simulink model "sampleModel184"  (R2021b)
settings: Solver=VariableStepAuto  StartTime=0.0  StopTime=10.0  RelTol=1e-3
libraries: simulink x11
settings Model: Creator=user  LastModifiedBy=user

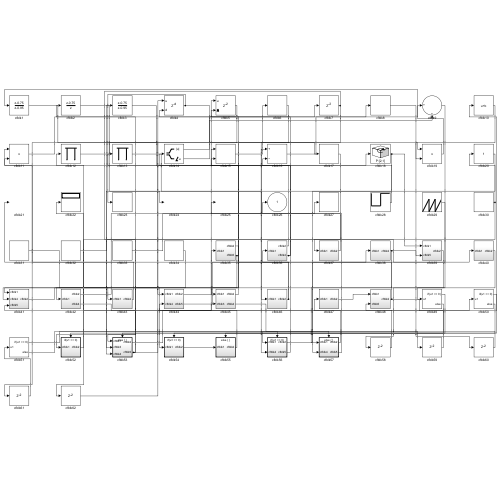
[thumbnail: Simulink's stored preview of the top-level diagram]
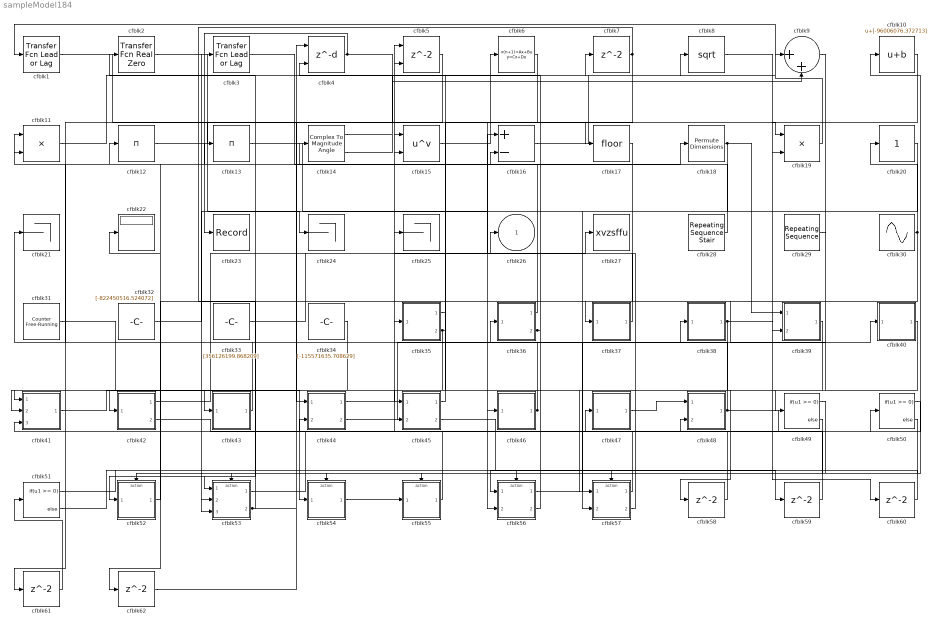
== system sampleModel184 ==
  cfblk1 : simulink/Discrete/Transfer Fcn Lead or Lag  PoleZ=0.95  ZeroZ=0.75  ICPrevOutput=0.0  ICPrevInput=0.0  DoSatur=off
      settings: SourceProductBaseCode=SL
  cfblk10 : Bias  Bias=[-96006076.372713]
  cfblk11 : Product  Inputs=**
  cfblk12 : Product  Inputs=*
  cfblk13 : Product  Inputs=*
  cfblk14 : ComplexToMagnitudeAngle
  cfblk15 : Math  Operator=pow  SaturateOnIntegerOverflow=on
  cfblk16 : Sum  Inputs=+-
  cfblk17 : Rounding
  cfblk18 : PermuteDimensions
  cfblk19 : Product
  cfblk2 : simulink/Discrete/Transfer Fcn Real Zero  ZeroZ=0.75  ICPrevInput=0.0  DoSatur=off
      settings: SourceProductBaseCode=SL
  cfblk20 : simulink/Math Operations/Slider Gain  gain=1  low=0  high=2
  cfblk21 : Terminator
  cfblk22 : Display
  cfblk23 : Record  FileSettingsInternal="{\"entries\":[{\"content\":{\"excelSettings\":{\"content\":{},\"type\":\"Streamout.ExcelSettings\"}},\"type\":\"Streamout.FileSettingStorage\",\"uuid\":\"3bb29845-961e-4fee-bd6d-4ce92e24b57c\"}],\"packageUris\":[\"http://schema.mathworks.com/mf0/streamout_blocks/R2020a\"],\"version\":\"1.0\"}"  SignalsInternal="{\"entries\":[{\"content\":{\"signals\":[{\"content\":{\"blockPath\":[\"sampleModel184/cfblk23\"],\"channel\":[],\"dimensions\":[1],\"domain\":\"sampleModel184/cfblk23\",\"lineColor\":\"#4dbeee\",\"plots\":[1],\"port\":1,\"sid\":[\"\"],\"signalID\":6859,\"signalName\":\"cfblk4\"},\"type\":\"RecordBlkView.Signal\",\"uuid\":\"63a490c9-4ba1-4137-91fe-6ad1500206e2\"}]},\"type\":\"RecordBlkView.InputSignals\",\"uuid\":\"3eea0c6d-d5bb-49b1-9db6-edc089c19657\"}],\"packageUris\":[\"http://schema.mathworks.com/mf0/streamout_blocks/R2020a\"],\"version\":\"1.0\"}"  VisualizationBindings="{\"sparklinesplugin\":{\"info\":[{\"bindingParametersList\":[],\"subplotID\":1}]}}"
  cfblk24 : Terminator
  cfblk25 : Terminator
  cfblk27 : ToWorkspace  VariableName=xvzsffu  SaveFormat=Timeseries  SampleTime=-1
  cfblk28 : simulink/Sources/Repeating Sequence Stair  OutValues=[100473429.883749, 716274051.172989]  tsamp=-1  OutMin=[]  OutMax=[]  OutDataTypeStr=double  OutputDataTypeScalingMode=double  OutDataType=fixdt(0,8)  ConRadixGroup=Best Precision: Vector-wise  OutScaling=2^-12
  cfblk29 : simulink/Sources/Repeating Sequence  rep_seq_t=[0 2]  rep_seq_y=[-291271804.102666, -101111727.446018]
  cfblk3 : simulink/Discrete/Transfer Fcn Lead or Lag  PoleZ=0.95  ZeroZ=0.75  ICPrevOutput=0.0  ICPrevInput=0.0  DoSatur=off
      settings: SourceProductBaseCode=SL
  cfblk30 : Sin  Amplitude=[486537178.471700]  Bias=[-87359593.712021]  SampleTime=0
  cfblk31 : simulink/Sources/Counter Free-Running  NumBits=[28.000000]  tsamp=-1
  cfblk32 : Constant  Value=[-822450516.524072]  SampleTime=1
  cfblk33 : Constant  Value=[356126199.868209]  SampleTime=1
  cfblk34 : Constant  Value=[-115571635.708629]  SampleTime=1
  cfblk35 : Subsystem
  cfblk36 : Subsystem
  cfblk37 : Subsystem
  cfblk38 : Subsystem
  cfblk39 : Subsystem
  cfblk4 : Delay  DelayLengthSource=Input port  SampleTime=1
      settings: InputPortMap=u0,p1
  cfblk40 : Subsystem
  cfblk41 : Subsystem
  cfblk42 : Subsystem
  cfblk43 : Subsystem
  cfblk44 : Subsystem
  cfblk45 : Subsystem
  cfblk46 : Subsystem
  cfblk47 : Subsystem
  cfblk48 : Subsystem
  cfblk49 : If  IfExpression=u1 >= 0  SampleTime=1
  cfblk5 : Delay  ShowEnablePort=on  SampleTime=1
      settings: InputPortMap=u0,e6
  cfblk50 : If  IfExpression=u1 >= 0  SampleTime=1
  cfblk51 : If  IfExpression=u1 >= 0  SampleTime=1
  cfblk52 : Subsystem  TreatAsAtomicUnit=on
  cfblk53 : Subsystem  TreatAsAtomicUnit=on
  cfblk54 : Subsystem  TreatAsAtomicUnit=on
  cfblk55 : Subsystem  TreatAsAtomicUnit=on
  cfblk56 : Subsystem  TreatAsAtomicUnit=on
  cfblk57 : Subsystem  TreatAsAtomicUnit=on
  cfblk{7,58..62} (6 alike) : Delay  SampleTime=1
  cfblk6 : DiscreteStateSpace
  cfblk8 : Sqrt  SaturateOnIntegerOverflow=on
  cfblk9 : Sum  Inputs=|++
  cfblk26 : Outport
  wires:
  cfblk43/1(cfblk2) -> cfblk21/1
  cfblk54/1(cfblk2) -> cfblk55/1(cfblk1)
  cfblk4/1 -> cfblk23/1, cfblk17/1
  cfblk3/1 -> cfblk18/1
  cfblk30/1 -> cfblk20/1, cfblk53/3(cfblk4)
  cfblk18/1 -> cfblk39/1(cfblk1), cfblk53/2(cfblk3)
  cfblk57/1(cfblk2) -> cfblk47/1(cfblk1)
  cfblk7/1 -> cfblk52/1(cfblk1), cfblk45/1(cfblk1)
  cfblk2/1 -> cfblk24/1
  cfblk40/1(cfblk2) -> cfblk57/1(cfblk1)
  cfblk15/1 -> cfblk6/1
  cfblk38/1(cfblk2) -> cfblk60/1, cfblk61/1
  cfblk9/1 -> cfblk37/1(cfblk1)
  cfblk35/1(cfblk2) -> cfblk42/1(cfblk1)
  cfblk42/1(cfblk2) -> cfblk27/1
  cfblk48/1(cfblk2) -> cfblk10/1, cfblk11/2
  cfblk37/1(cfblk2) -> cfblk26/1
  cfblk56/1(cfblk2) -> cfblk38/1(cfblk1)
  cfblk44/1(cfblk2) -> cfblk5/1
  cfblk31/1 -> cfblk54/1(cfblk1)
  cfblk13/1 -> cfblk46/1(cfblk1)
  cfblk55/1(cfblk2) -> cfblk12/1
  cfblk12/1 -> cfblk19/1
  cfblk32/1 -> cfblk3/1
  cfblk52/1(cfblk2) -> cfblk22/1
  cfblk20/1 -> cfblk57/2(cfblk4)
  cfblk6/1 -> cfblk56/2(cfblk4)
  cfblk56/2(cfblk5) -> cfblk4/2
  cfblk41/1(cfblk2) -> cfblk43/1(cfblk1)
  cfblk8/1 -> cfblk19/2
  cfblk1/1 -> cfblk44/1(cfblk1)
  cfblk47/1(cfblk2) -> cfblk48/1(cfblk1)
  cfblk11/1 -> cfblk7/1
  cfblk19/1 -> cfblk1/1
  cfblk29/1 -> cfblk49/1
  cfblk42/2(cfblk4) -> cfblk50/1
  cfblk53/1(cfblk2) -> cfblk35/1(cfblk1)
  cfblk57/2(cfblk5) -> cfblk25/1
  cfblk33/1 -> cfblk16/1
  cfblk45/1(cfblk2) -> cfblk5/2
  cfblk16/1 -> cfblk8/1
  cfblk28/1 -> cfblk13/1
  cfblk35/2(cfblk5) -> cfblk15/1, cfblk41/2(cfblk4)
  cfblk34/1 -> cfblk53/1(cfblk1)
  cfblk53/2(cfblk5) -> cfblk2/1, cfblk41/3(cfblk5), cfblk45/2(cfblk3)
  cfblk10/1 -> cfblk39/2(cfblk5)
  cfblk46/1(cfblk2) -> cfblk36/1(cfblk1), cfblk15/2
  cfblk36/1(cfblk2) -> cfblk14/1
  cfblk44/2(cfblk5) -> cfblk40/1(cfblk1)
  cfblk36/2(cfblk4) -> cfblk16/2, cfblk11/1
  cfblk14/1 -> cfblk9/1
  cfblk5/1 -> cfblk41/1(cfblk1)
  cfblk14/2 -> cfblk9/2
  cfblk49/1 -> cfblk52/Action
  cfblk49/2 -> cfblk53/Action
  cfblk50/1 -> cfblk54/Action
  cfblk50/2 -> cfblk55/Action
  cfblk51/1 -> cfblk56/Action
  cfblk51/2 -> cfblk57/Action
  cfblk39/1(cfblk2) -> cfblk58/1
  cfblk58/1 -> cfblk48/2(cfblk5)
  cfblk45/2(cfblk4) -> cfblk59/1
  cfblk59/1 -> cfblk44/2(cfblk4)
  cfblk60/1 -> cfblk56/1(cfblk1)
  cfblk61/1 -> cfblk51/1
  cfblk17/1 -> cfblk62/1
  cfblk62/1 -> cfblk4/1

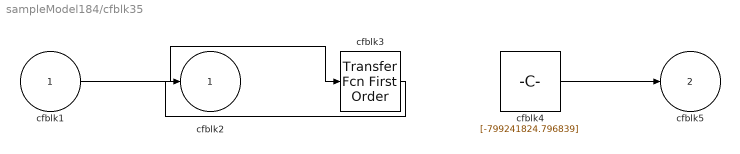
== system sampleModel184/cfblk35 ==
  cfblk1 : Inport
  cfblk3 : simulink/Discrete/Transfer Fcn First Order  PoleZ=0.95  ICPrevOutput=0.0  DoSatur=off
  cfblk4 : Constant  Value=[-799241824.796839]  SampleTime=1
  cfblk2 : Outport
  cfblk5 : Outport  Port=2
  wires:
  cfblk1/1 -> cfblk3/1
  cfblk4/1 -> cfblk5/1
  cfblk3/1 -> cfblk2/1

== system sampleModel184/cfblk36 ==
  cfblk1 : Inport
  cfblk3 : Assignment  DiagnosticForDimensions=Warning  IndexOptions=Index vector (dialog)  Indices=1  OutputSizes=1
  cfblk2 : Outport
  cfblk4 : Outport  Port=2
  wires:
  cfblk1/1 -> cfblk2/1, cfblk3/1, cfblk3/2
  cfblk3/1 -> cfblk4/1

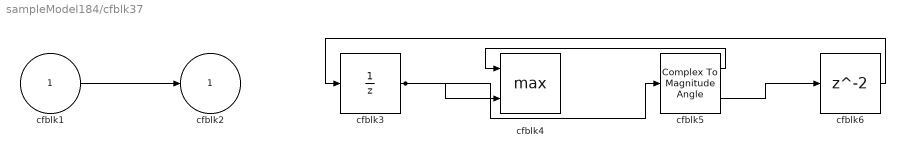
== system sampleModel184/cfblk37 ==
  cfblk1 : Inport
  cfblk3 : UnitDelay  HasFrameUpgradeWarning=on
  cfblk4 : MinMax  Function=max  Inputs=2
  cfblk5 : ComplexToMagnitudeAngle
  cfblk6 : Delay  SampleTime=1
  cfblk2 : Outport
  wires:
  cfblk1/1 -> cfblk2/1
  cfblk5/1 -> cfblk4/1
  cfblk3/1 -> cfblk5/1, cfblk4/2
  cfblk5/2 -> cfblk6/1
  cfblk6/1 -> cfblk3/1

== system sampleModel184/cfblk38 ==
  cfblk1 : Inport
  cfblk3 : ComplexToMagnitudeAngle
  cfblk4 : Bias  Bias=[821146582.759653]
  cfblk2 : Outport
  wires:
  cfblk3/1 -> cfblk2/1
  cfblk1/1 -> cfblk4/1
  cfblk4/1 -> cfblk3/1

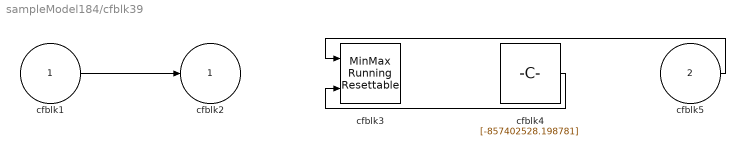
== system sampleModel184/cfblk39 ==
  cfblk1 : Inport
  cfblk5 : Inport  Port=2
  cfblk3 : simulink/Math Operations/MinMax Running Resettable  Function=min  vinit=0.0
  cfblk4 : Constant  Value=[-857402528.198781]  SampleTime=1
  cfblk2 : Outport
  wires:
  cfblk1/1 -> cfblk2/1
  cfblk5/1 -> cfblk3/1
  cfblk4/1 -> cfblk3/2

== system sampleModel184/cfblk40 ==
  cfblk1 : Inport
  cfblk3 : Constant  Value=[639037280.351687]  SampleTime=1
  cfblk2 : Outport
  wires:
  cfblk1/1 -> cfblk2/1

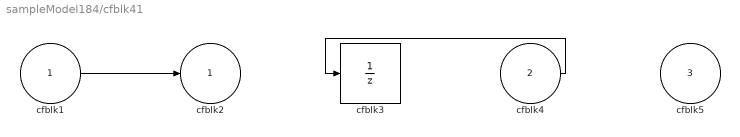
== system sampleModel184/cfblk41 ==
  cfblk1 : Inport
  cfblk4 : Inport  Port=2
  cfblk5 : Inport  Port=3
  cfblk3 : UnitDelay  HasFrameUpgradeWarning=on
  cfblk2 : Outport
  wires:
  cfblk1/1 -> cfblk2/1
  cfblk4/1 -> cfblk3/1

== system sampleModel184/cfblk42 ==
  cfblk1 : Inport
  cfblk3 : Sqrt  SaturateOnIntegerOverflow=on
  cfblk2 : Outport
  cfblk4 : Outport  Port=2
  wires:
  cfblk1/1 -> cfblk3/1
  cfblk3/1 -> cfblk2/1, cfblk4/1

== system sampleModel184/cfblk43 ==
  cfblk1 : Inport
  cfblk3 : Delay  DelayLengthSource=Input port  SampleTime=1
      settings: InputPortMap=u0,p1
  cfblk2 : Outport
  wires:
  cfblk1/1 -> cfblk3/1, cfblk3/2
  cfblk3/1 -> cfblk2/1

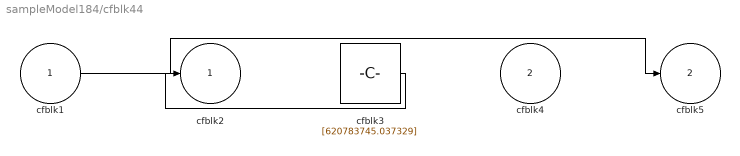
== system sampleModel184/cfblk44 ==
  cfblk1 : Inport
  cfblk4 : Inport  Port=2
  cfblk3 : Constant  Value=[620783745.037329]  SampleTime=1
  cfblk2 : Outport
  cfblk5 : Outport  Port=2
  wires:
  cfblk1/1 -> cfblk5/1
  cfblk3/1 -> cfblk2/1

== system sampleModel184/cfblk45 ==
  cfblk1 : Inport
  cfblk3 : Inport  Port=2
  cfblk2 : Outport
  cfblk4 : Outport  Port=2
  wires:
  cfblk3/1 -> cfblk2/1
  cfblk1/1 -> cfblk4/1

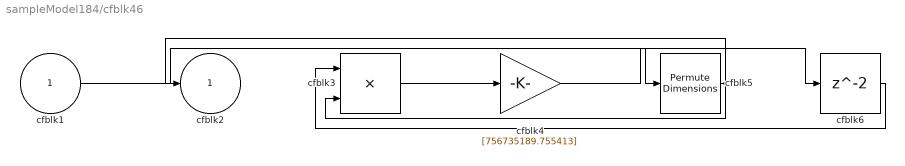
== system sampleModel184/cfblk46 ==
  cfblk1 : Inport
  cfblk3 : Product
  cfblk4 : Gain  Gain=[756735189.755413]
  cfblk5 : PermuteDimensions
  cfblk6 : Delay  SampleTime=1
  cfblk2 : Outport
  wires:
  cfblk1/1 -> cfblk5/1
  cfblk5/1 -> cfblk2/1, cfblk3/2
  cfblk3/1 -> cfblk4/1
  cfblk4/1 -> cfblk6/1
  cfblk6/1 -> cfblk3/1

== system sampleModel184/cfblk47 ==
  cfblk1 : Inport
  cfblk3 : Sum  Inputs=|++
  cfblk4 : Constant  Value=[657642425.472203]  SampleTime=1
  cfblk2 : Outport
  wires:
  cfblk3/1 -> cfblk2/1
  cfblk1/1 -> cfblk3/1
  cfblk4/1 -> cfblk3/2

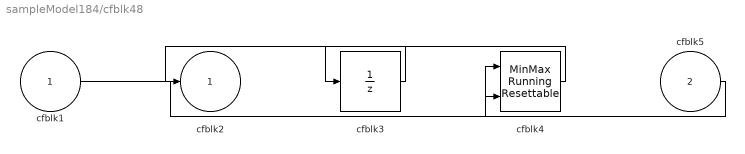
== system sampleModel184/cfblk48 ==
  cfblk1 : Inport
  cfblk5 : Inport  Port=2
  cfblk3 : UnitDelay  HasFrameUpgradeWarning=on
  cfblk4 : simulink/Math Operations/MinMax Running Resettable  Function=min  vinit=0.0
  cfblk2 : Outport
  wires:
  cfblk4/1 -> cfblk3/1
  cfblk1/1 -> cfblk4/1
  cfblk3/1 -> cfblk2/1
  cfblk5/1 -> cfblk4/2

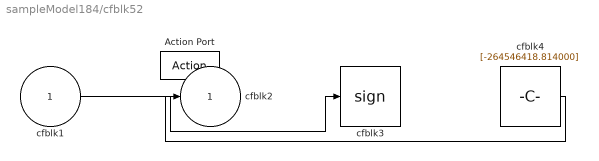
== system sampleModel184/cfblk52 ==
  cfblk1 : Inport
  Action Port : ActionPort  ActionPortLabel=if(u1 >= 0)
  cfblk3 : Signum
  cfblk4 : Constant  Value=[-264546418.814000]  SampleTime=1
  cfblk2 : Outport
  wires:
  cfblk1/1 -> cfblk3/1
  cfblk4/1 -> cfblk2/1

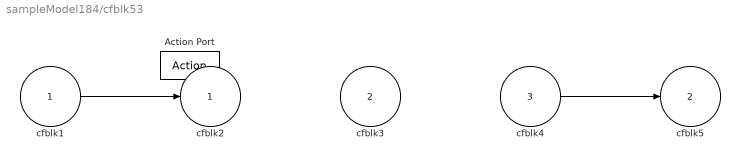
== system sampleModel184/cfblk53 ==
  cfblk1 : Inport
  cfblk3 : Inport  Port=2
  cfblk4 : Inport  Port=3
  Action Port : ActionPort  ActionPortLabel=else
  cfblk2 : Outport
  cfblk5 : Outport  Port=2
  wires:
  cfblk4/1 -> cfblk5/1
  cfblk1/1 -> cfblk2/1

== system sampleModel184/cfblk54 ==
  cfblk1 : Inport
  Action Port : ActionPort  ActionPortLabel=if(u1 >= 0)
  cfblk3 : Sum  Inputs=-+
  cfblk4 : Constant  Value=[-583830235.402709]  SampleTime=1
  cfblk2 : Outport
  wires:
  cfblk3/1 -> cfblk2/1
  cfblk4/1 -> cfblk3/1
  cfblk1/1 -> cfblk3/2

== system sampleModel184/cfblk55 ==
  cfblk1 : Inport
  Action Port : ActionPort  ActionPortLabel=else
  cfblk3 : simulink/Discrete/Transfer Fcn Lead or Lag  PoleZ=0.95  ZeroZ=0.75  ICPrevOutput=0.0  ICPrevInput=0.0  DoSatur=off
      settings: SourceProductBaseCode=SL
  cfblk4 : Constant  Value=[487504683.906193]  SampleTime=1
  cfblk2 : Outport
  wires:
  cfblk4/1 -> cfblk2/1
  cfblk1/1 -> cfblk3/1

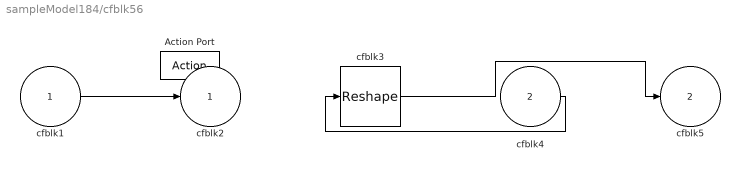
== system sampleModel184/cfblk56 ==
  cfblk1 : Inport
  cfblk4 : Inport  Port=2
  Action Port : ActionPort  ActionPortLabel=if(u1 >= 0)
  cfblk3 : Reshape
  cfblk2 : Outport
  cfblk5 : Outport  Port=2
  wires:
  cfblk3/1 -> cfblk5/1
  cfblk1/1 -> cfblk2/1
  cfblk4/1 -> cfblk3/1

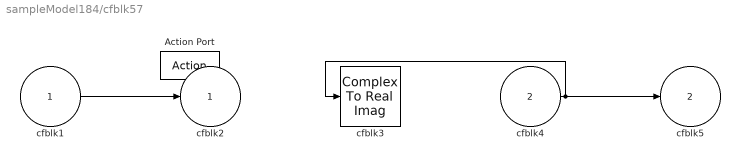
== system sampleModel184/cfblk57 ==
  cfblk1 : Inport
  cfblk4 : Inport  Port=2
  Action Port : ActionPort  ActionPortLabel=else
  cfblk3 : ComplexToRealImag
  cfblk2 : Outport
  cfblk5 : Outport  Port=2
  wires:
  cfblk4/1 -> cfblk5/1, cfblk3/1
  cfblk1/1 -> cfblk2/1
